simulink model "Linear_ADMIRE_sim"  (Simulink 8.4)
settings: Solver=ode4  StartTime=0.0  StopTime=10  FixedStep=dt  RelTol=1e-3
InitFcn:
  | INIT_LINEAR
values from neighbouring files (symbols this model uses):
  a1 = (180*d2r)/(80^3)    (= 6.13592315154e-06)    [INIT_LINEAR.m]    (also in INIT_NDI.m)
  a2 = (24*d2r)/(80^3)    (= 8.18123086872e-07)    [INIT_LINEAR.m]    (also in INIT_NDI.m)
  a3 = (5*d2r)/(200)    (= 0.000436332312999)    [INIT_LINEAR.m]    (also in INIT_NDI.m)
  Abare = [-0.0369710265542 -0.00338320638614 0 0 0.00101076287488 0 0 0 0 1.00000000002 0 1.7763568394e-12 ... (784 elements, 28x28)]    [Trim_M0p22ALT20_LinDATA.mat]    (also in Trim_M0p3ALT2000_LinDATA.mat = [-0.0208061645292 -0.00191640084378 0 0 0.000610808752105 0 )
  Bbare = [-1.10043807057 0.00182125944543 -0.00701366565749 0.707306131876 1.12037014439 -0.330899025785 0 0 0 0 0 0 ... (448 elements, 28x16)]    [Trim_M0p22ALT20_LinDATA.mat]    (also in Trim_M0p3ALT2000_LinDATA.mat = [-1.42042676365 -0.000549876720984 -0.00633411409606 0.84954)
  CAmethod = 1    [ACA_init.m]    (also in INIT_LINEAR.m = 0; INIT_NDI.m = 0)
  Canard_max = interp1(M_vec,[25 25 25 15 15 15 15 15]*d2r,Mach,'next')    [INIT_LINEAR.m]    (also in INIT_NDI.m = [25 25 25 15 15 15 15 15]*d2r)
  Canard_min = interp1(M_vec,[-55 -55 -25 -15 -15 -15 -15 -15]*d2r,Mach,'next')    [INIT_LINEAR.m]    (also in INIT_NDI.m = [-55 -55 -25 -15 -15 -15 -15 -15]*d2r)
  CAobm = CAobm(:,1:12)    [INIT_LINEAR.m]
  Cbare = [1 0 0 0 0 0 0 0 0 0 0 0 ... (1652 elements, 59x28)]    [Trim_M0p22ALT20_LinDATA.mat]    (also in Trim_M0p3ALT2000_LinDATA.mat)
  CBobm = CCV*Bbare    [INIT_LINEAR.m]
  Dbare = [0 0 0 0 0 0 0 0 0 0 0 0 ... (944 elements, 59x16)]    [Trim_M0p22ALT20_LinDATA.mat]    (also in Trim_M0p3ALT2000_LinDATA.mat)
  dt = 0.01    [ACA_init.m]    (also in INIT_LINEAR.m; INIT_NDI.m)
  DTY_max = 0.002    [ACA_init.m]    (also in INIT_LINEAR.m; INIT_NDI.m)
  DTY_min = -0.002    [ACA_init.m]    (also in INIT_LINEAR.m; INIT_NDI.m)
  DTZ_max = 0.002    [ACA_init.m]    (also in INIT_LINEAR.m; INIT_NDI.m)
  DTZ_min = -0.002    [ACA_init.m]    (also in INIT_LINEAR.m; INIT_NDI.m)
  Elevon_max = interp1(M_vec,[30 30 25 25 25 25 25 25]*d2r,Mach,'next')    [INIT_LINEAR.m]    (also in INIT_NDI.m = [30 30 25 25 25 25 25 25]*d2r)
  Elevon_min = interp1(M_vec,[-30 -30 -30 -30 -30 -30 -30 -30]*d2r,Mach,'next')    [INIT_LINEAR.m]    (also in INIT_NDI.m = [-30 -30 -30 -30 -30 -30 -30 -30]*d2r)
  Fas_t = [0 1 1+dt 2. 2.+dt 8]    [INIT_LINEAR.m]
  Fas_v = [0 0 1 1 0 0]*40*0    [INIT_LINEAR.m]
  Fes_t = [0 1 1+dt 4 4+dt 7 7+dt 8]    [INIT_LINEAR.m]
  Fes_v = [0 0 1 1 -1 -1 0 0]*40    [INIT_LINEAR.m]
  Frp_t = [0 1 1+dt 6. 6.+dt 8]    [INIT_LINEAR.m]
  Frp_v = [0 0 1 1 0 0]*100*0    [INIT_LINEAR.m]
  G = [ 0 1 0 ... (first row only)    [ACA_init.m]    (also in INIT_LINEAR.m = [ 1 0 0; INIT_NDI.m)
  Kfb = -1.71    [INIT_LINEAR.m]
  Kfq = -3.4    [INIT_LINEAR.m]
  Kib = 5.14    [INIT_LINEAR.m]
  Kiq = 4    [INIT_LINEAR.m]
  Kp = 2.    (= 2)    [INIT_LINEAR.m]
  Kpb = 4.29    [INIT_LINEAR.m]
  Kpq = 3.4    [INIT_LINEAR.m]
  Kr = 14    [INIT_LINEAR.m]
  LEF_max = interp1(M_vec,[30 30 30 20 20 15 10 10]*d2r,Mach,'next')    [INIT_LINEAR.m]    (also in INIT_NDI.m = [30 30 30 20 20 15 10 10]*d2r)
  LEF_min = interp1(M_vec,[-10 -10 -10 -10 -10 -10 -10 -10]*d2r,Mach,'next')    [INIT_LINEAR.m]    (also in INIT_NDI.m = [-10 -10 -10 -10 -10 -10 -10 -10]*d2r)
  LG_max = 1    [ACA_init.m]    (also in INIT_LINEAR.m; INIT_NDI.m)
  LG_min = 0    [ACA_init.m]    (also in INIT_LINEAR.m; INIT_NDI.m)
  LPmethod = 3    [ACA_init.m]    (also in INIT_LINEAR.m = 0; INIT_NDI.m = 0; LPwrap.m = 0; LPwrap_1.m = 0)
  NumU = 16    [ACA_init.m]    (also in INIT_LINEAR.m; INIT_NDI.m; test.m; test_LPwrap.m)
  PD_max = 10    [ACA_init.m]    (also in INIT_LINEAR.m; INIT_NDI.m)
  PD_min = -10    [ACA_init.m]    (also in INIT_LINEAR.m; INIT_NDI.m)
  r2d = 180/pi    (= 57.2957795131)    [ACA_init.m]    (also in INIT_LINEAR.m; INIT_NDI.m)
  Rudder_max = interp1(M_vec,[30 30 25 20 15 15 15 10]*d2r,Mach,'next')    [INIT_LINEAR.m]    (also in INIT_NDI.m = [30 30 25 20 15 15 15 10]*d2r)
  Rudder_min = interp1(M_vec,[-30 -30 -25 -20 -15 -15 -15 -10]*d2r,Mach,'next')    [INIT_LINEAR.m]    (also in INIT_NDI.m = [-30 -30 -25 -20 -15 -15 -15 -10]*d2r)
  TSS_max = 1    [ACA_init.m]    (also in INIT_LINEAR.m; INIT_NDI.m)
  TSS_min = 0    [ACA_init.m]    (also in INIT_LINEAR.m; INIT_NDI.m)
  TSS_t = [0 1 1+dt 6. 6.+dt 8]    [INIT_LINEAR.m]
  TSS_v = [0 0 .1 .1 0 0]*0+u0new(10)    [INIT_LINEAR.m]
  UACTIVE = [ ... (first row only)    [INIT_LINEAR.m]
  UD_max = 10    [ACA_init.m]    (also in INIT_LINEAR.m; INIT_NDI.m)
  UD_min = -10    [ACA_init.m]    (also in INIT_LINEAR.m; INIT_NDI.m)
  Umax = [Canard_max*[1 1] Elevon_max*[1 1 1 1] Rudder_max LEF_max     LG_max TSS_max DTY_max DTZ_max UD_max VD_max WD_max PD_max]'    [INIT_LINEAR.m]    (also in INIT_NDI.m = [25 25 30 30 30 30 30]'*d2r)
  Umin = [Canard_min*[1 1] Elevon_min*[1 1 1 1] Rudder_min LEF_min     LG_min TSS_min DTY_min DTZ_min UD_min VD_min WD_min PD_min]'    [INIT_LINEAR.m]    (also in INIT_NDI.m = [-55 -55 -30 -30 -30 -30 -30]'*d2r)
  Unom = u0new    [INIT_LINEAR.m]
  Upref = [0 0 0 0 0 0 0 0 0 0 0 0 0 0 0 0]'    [ACA_init.m]    (also in INIT_LINEAR.m; INIT_NDI.m)
  UsePref = 0    [INIT_LINEAR.m]
  VD_max = 10    [ACA_init.m]    (also in INIT_LINEAR.m; INIT_NDI.m)
  VD_min = -10    [ACA_init.m]    (also in INIT_LINEAR.m; INIT_NDI.m)
  WD_max = 10    [ACA_init.m]    (also in INIT_LINEAR.m; INIT_NDI.m)
  WD_min = -10    [ACA_init.m]    (also in INIT_LINEAR.m; INIT_NDI.m)
  Wp = W'*W    [ACA_init.m]    (also in INIT_LINEAR.m; INIT_NDI.m; test.m; test_LPwrap.m)
  y0bare = [74.8477877145 0.159877852888 0 0 0 0 0 0.159877852888 0 0 0 -20 ... (73 elements, 73x1)]    [Trim_M0p22ALT20_LinDATA.mat]    (also in Trim_M0p3ALT2000_LinDATA.mat = [99.7587452043 0.116024082006 0 0 0 0 0 0.116024082006 0 0 0)
undefined symbols (not defined in the file or in its folder): CGIwrap, DAwrap, LPwrap, VJAwrap
libraries: simulink x6
(part 2 of 2)

== system Linear_ADMIRE_sim/ControlAllocation/GetU/WeightedPseudo Scaled_2/Blocks/Some_Saturated/For Iterator Subsystem/If Action Subsystem1/If Action Subsystem ==
  u : Inport
  ulim : Inport  Port=2
  scale_z : Inport  Port=3
  Action Port : ActionPort  ActionType=then
  MinMax : MinMax  Inputs=2
  Product : Product  Inputs=*/  RndMeth=Zero
  Out1 : Outport
  wires:
  MinMax/1 -> Out1/1
  Product/1 -> MinMax/1
  u/1 -> Product/2
  ulim/1 -> Product/1
  scale_z/1 -> MinMax/2

== system Linear_ADMIRE_sim/ControlAllocation/GetU/WeightedPseudo Scaled_2/Blocks/Some_Saturated/For Iterator Subsystem/If Action Subsystem1/If Action Subsystem1 ==
  Action Port : ActionPort  ActionType=else
  Constant4 : Constant  Value=0
  Out1 : Outport
  wires:
  Constant4/1 -> Out1/1

== system Linear_ADMIRE_sim/ControlAllocation/GetU/WeightedPseudo Scaled_2/Blocks/Some_Saturated/For Iterator Subsystem/If Action Subsystem2/If Action Subsystem ==
  u : Inport
  ulim : Inport  Port=2
  scale_z : Inport  Port=3
  Action Port : ActionPort  ActionType=then
  MinMax : MinMax  Inputs=2
  Product : Product  Inputs=*/  RndMeth=Zero
  Out1 : Outport
  wires:
  MinMax/1 -> Out1/1
  Product/1 -> MinMax/1
  u/1 -> Product/2
  ulim/1 -> Product/1
  scale_z/1 -> MinMax/2

== system Linear_ADMIRE_sim/ControlAllocation/GetU/WeightedPseudo Scaled_2/Blocks/Some_Saturated/For Iterator Subsystem/If Action Subsystem2/If Action Subsystem1 ==
  Action Port : ActionPort  ActionType=else
  Constant4 : Constant  Value=0
  Out1 : Outport
  wires:
  Constant4/1 -> Out1/1
